simulink model "DPendulum_Simple"  (R2023a)
settings: Solver=VariableStepAuto  StartTime=0.0  StopTime=10  RelTol=1e-3
settings Model: Creator=Inovicht  LastModifiedBy=Inovicht

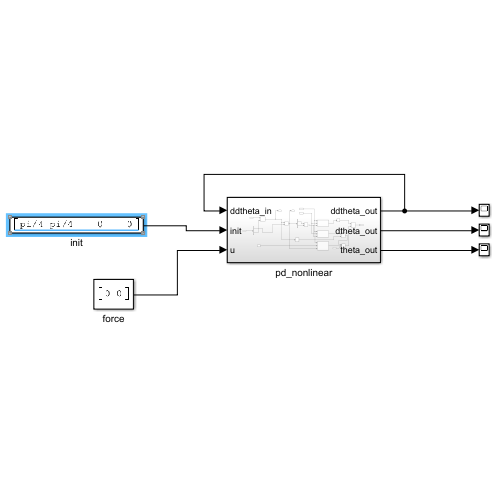
[thumbnail: Simulink's stored preview of the top-level diagram]
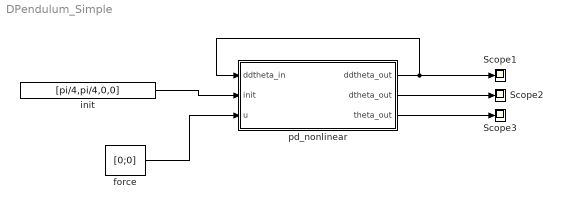
== system DPendulum_Simple ==
  Scope1 : Scope
  Scope2 : Scope
  Scope3 : Scope
  force : Constant  Value=[0;0]
  init : Constant  Value=[pi/4,pi/4,0,0]
  pd_nonlinear : Subsystem
  wires:
  force/1 -> pd_nonlinear/3(u)
  pd_nonlinear/1(ddtheta_out) -> pd_nonlinear/1(ddtheta_in), Scope1/1
  init/1 -> pd_nonlinear/2(init)
  pd_nonlinear/2(dtheta_out) -> Scope2/1
  pd_nonlinear/3(theta_out) -> Scope3/1

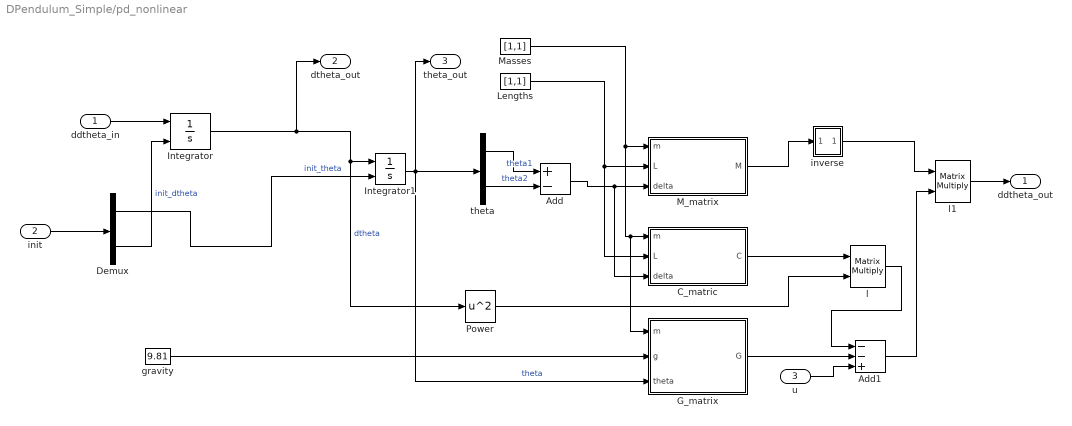
== system DPendulum_Simple/pd_nonlinear ==
  ddtheta_in : Inport  PortDimensions=2
  init : Inport  Port=2  PortDimensions=4
  u : Inport  Port=3  PortDimensions=2
  Add : Sum  Inputs=+-
  Add1 : Sum  Inputs=--+
  C_matric : MATLAB Function  TreatAsAtomicUnit=on
  Demux : Demux  Outputs=[2 2]
  G_matrix : MATLAB Function  TreatAsAtomicUnit=on
  Integrator : Integrator  InitialConditionSource=external
  Integrator1 : Integrator  InitialConditionSource=external
  Lengths : Constant  Value=[1,1]
  M_matrix : MATLAB Function  TreatAsAtomicUnit=on
  Masses : Constant  Value=[1,1]
  Power : Math  Operator=square
  gravity : Constant  Value=9.81
  inverse : MATLAB Function  TreatAsAtomicUnit=on
  l : Product  Multiplication=Matrix(*)
  l1 : Product  Multiplication=Matrix(*)
  theta : Demux  Outputs=2
  ddtheta_out : Outport
  dtheta_out : Outport  Port=2
  theta_out : Outport  Port=3
  wires:
  l/1 -> Add1/1
  inverse/1(A_inv) -> l1/1
  M_matrix/1(M) -> inverse/1(A)
  C_matric/1(C) -> l/1
  ddtheta_in/1 -> Integrator/1
  G_matrix/1(G) -> Add1/2
  u/1 -> Add1/3
  init/1 -> Demux/1
  Add1/1 -> l1/2
  Integrator/1 -> Power/1, Integrator1/1, dtheta_out/1  "dtheta"
  l1/1 -> ddtheta_out/1
  Demux/2 -> Integrator/2  "init_dtheta"
  Demux/1 -> Integrator1/2  "init_theta"
  theta/2 -> Add/2  "theta2"
  theta/1 -> Add/1  "theta1"
  Masses/1 -> G_matrix/1(m), C_matric/1(m), M_matrix/1(m)
  Lengths/1 -> C_matric/2(L), M_matrix/2(L)
  gravity/1 -> G_matrix/2(g)
  Add/1 -> C_matric/3(delta), M_matrix/3(delta)
  Power/1 -> l/2
  Integrator1/1 -> G_matrix/3(theta), theta_out/1, theta/1  "theta"

== matlab function DPendulum_Simple/pd_nonlinear/C_matric ==
  data: m input; L input; C output; delta input
function C = C_matrix(m,L,delta)
m2 = m(2);
m1 = m(1);
l1 = L(1);
l2 = L(2);

C = [0, m2*l2*sin(delta); l1*sin(delta)  , 0];  % Coupling matrix
end

== matlab function DPendulum_Simple/pd_nonlinear/G_matrix ==
  data: m input; g input; G output; theta input
function G = G_matrix(m,g,theta)
m2 = m(2);
m1 = m(1);
g = g;
theta_1 = theta(1);
theta_2 = theta(2);
G = [(m1+m2)*g*sin(theta_1); g*sin(theta_2)];                 % Gravitational matrix
end

== matlab function DPendulum_Simple/pd_nonlinear/M_matrix ==
  data: m input; L input; delta input; M output
function M  = M_matrix(m,L,delta)
m2 = m(2);
m1 = m(1);
l1 = L(1);
l2 = L(2);
M = [(m1+m2)*l1  , m2*l2*cos(delta); l1*cos(delta)  , l2]; % Mass matrix
end

== matlab function DPendulum_Simple/pd_nonlinear/inverse ==
  data: A input; A_inv output
function A_inv = fcn(A)
    A_inv = inv(A);
end
